simulink model "untitled"  (R2015b)
settings: Solver=VariableStepAuto  StartTime=0.0  StopTime=300  RelTol=1e-3
libraries: simulink_extras x1, fl_lib x1, powerlib_meascontrol x1
settings Model: Creator=Bogdan.Borowy  LastModifiedBy=Bogdan.Borowy

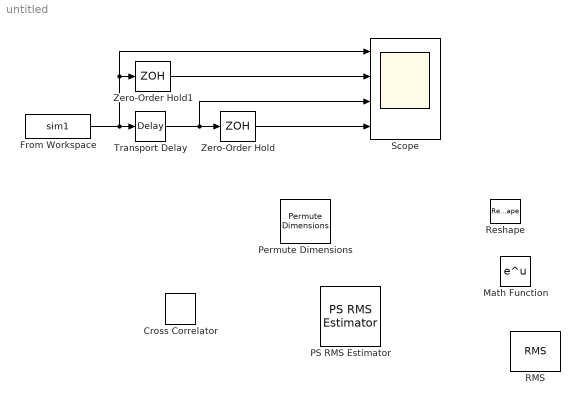
== system untitled ==
  Cross Correlator : simulink_extras/Additional Sinks/Cross Correlator  npts=100  HowOften=50  sampleT=0.1
  From Workspace : FromWorkspace  VariableName=sim1  SampleTime=0  OutputAfterFinalValue=Setting to zero
  Math Function : Math  SaturateOnIntegerOverflow=on
  PS RMS Estimator : fl_lib/Physical Signals/Periodic Operators/PS RMS Estimator  f0=60 Hz
  Permute Dimensions : PermuteDimensions
  RMS : powerlib_meascontrol/Measurements/RMS  TrueRMS=on  Freq=60  RMSInit=120  Ts=0
  Reshape : Reshape
  Scope : Scope  NumInputPorts=4
  Transport Delay : TransportDelay  DelayTime=10
  Zero-Order Hold : ZeroOrderHold  SampleTime=10
  Zero-Order Hold1 : ZeroOrderHold  SampleTime=10
  wires:
  From Workspace/1 -> Scope/1, Zero-Order Hold1/1, Transport Delay/1
  Transport Delay/1 -> Scope/3, Zero-Order Hold/1
  Zero-Order Hold1/1 -> Scope/2
  Zero-Order Hold/1 -> Scope/4
